simulink model "IBVShandcoded"  (Simulink 5.0)
settings: Solver=ode45  StartTime=0.0  StopTime=30.0  RelTol=1e-3
values from neighbouring files (symbols this model uses):
  c = camera(1000,1000,256,256,512,512)    [initHBVS.m]    (also in vsbrowser.m = handles.c)
  p = reshape(u,2,n)    [CamView.m]    (also in initHBVS.m = polyhedra([0.0 0.0 0; 0.25 0.25 0; -0.25 0.25 0; -0.25 -0.25; vsbrowser.m = handles.p)
  T0c_0 = T0c    [initHBVS.m]
  T0c_x = T0c    [initHBVS.m]
  T0o = handles.T0o    [vsbrowser.m]
undefined symbols (not defined in the file or in its folder): coords, get, GetHMatrix
libraries: vs x10
settings Model: LastModifiedBy=ecervera  BooleanDataType=off

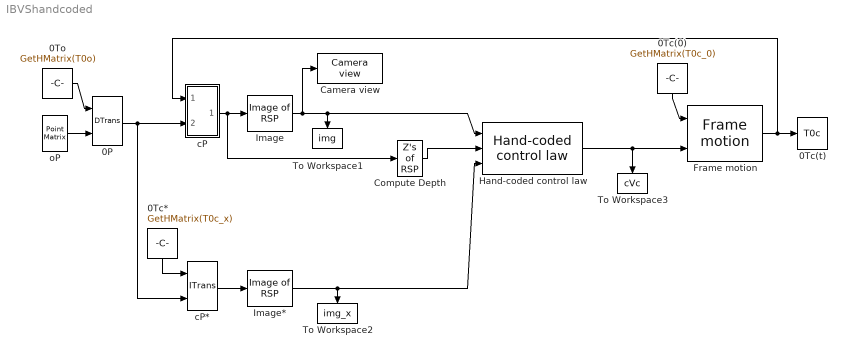
== system IBVShandcoded ==
  0P : vs/Features/DTrans  SimViewingDevice=off  DataTypeOverride=UseLocalSettings  MinMaxOverflowLogging=UseLocalSettings
      settings: Permissions=ReadWrite  RTWFcnNameOpts=Auto  RTWFileNameOpts=Auto
  0Tc(0) : Constant  Orientation=down  Value=GetHMatrix(T0c_0)  VectorParams1D=off
  0Tc(t) : ToWorkspace  VariableName=T0c  SampleTime=-1  SaveFormat=StructureWithTime
  0Tc* : Constant  Orientation=down  Value=GetHMatrix(T0c_x)  VectorParams1D=off
  0To : Constant  Value=GetHMatrix(T0o)  VectorParams1D=off
  Camera view : vs/Camera/Camera view  ms=15  em=normal  umin=0  umax=get(c,'hres')-1  vmin=0  vmax=get(c,'vres')-1  st=-1
  Compute Depth : vs/Features/Z's of RSP  SimViewingDevice=off  DataTypeOverride=UseLocalSettings  MinMaxOverflowLogging=UseLocalSettings
      settings: Permissions=ReadWrite  RTWFcnNameOpts=Auto  RTWFileNameOpts=Auto
  Frame motion : vs/Pose/Frame motion  SimViewingDevice=off  DataTypeOverride=UseLocalSettings  MinMaxOverflowLogging=UseLocalSettings
      settings: Permissions=ReadWrite  RTWFcnNameOpts=Auto  RTWFileNameOpts=Auto
  Hand-coded control law : vs/Jacobian/Hand-coded control law  n=size(coords(p),2)  fu=get(c,'fu')  fv=get(c,'fv')  u0=get(c,'u0')  v0=get(c,'v0')  lambda=lambda
  Image : vs/Camera/Image of RSP  fu=get(c,'fu')  fv=get(c,'fv')  u0=get(c,'u0')  v0=get(c,'v0')
  Image* : vs/Camera/Image of RSP  fu=get(c,'fu')  fv=get(c,'fv')  u0=get(c,'u0')  v0=get(c,'v0')
  To Workspace1 : ToWorkspace  VariableName=img  SampleTime=-1  SaveFormat=StructureWithTime
      settings: Orientation=down
  To Workspace2 : ToWorkspace  VariableName=img_x  SampleTime=-1  SaveFormat=StructureWithTime
      settings: Orientation=down
  To Workspace3 : ToWorkspace  VariableName=cVc  SampleTime=-1  SaveFormat=StructureWithTime
      settings: Orientation=down
  cP : Subsystem  AncestorBlock=vs/Features/ITrans
  cP* : vs/Features/ITrans  SimViewingDevice=off  DataTypeOverride=UseLocalSettings  MinMaxOverflowLogging=UseLocalSettings
      settings: Permissions=ReadWrite  RTWFcnNameOpts=Auto  RTWFileNameOpts=Auto
  oP : vs/Features/Point Matrix  m=coords(p)
  wires:
  oP/1 -> 0P/2
  cP/1(bP) -> Image/1, Compute Depth/1
  Image/1 -> Camera view/1, Hand-coded control law/1, To Workspace1/1
  Frame motion/1 -> 0Tc(t)/1, cP/1(aTb)
  0Tc*/1 -> cP*/1
  cP*/1 -> Image*/1
  Image*/1 -> Hand-coded control law/3, To Workspace2/1
  0Tc(0)/1 -> Frame motion/1
  0To/1 -> 0P/1
  0P/1 -> cP/2(aP), cP*/2
  Hand-coded control law/1 -> To Workspace3/1, Frame motion/2
  Compute Depth/1 -> Hand-coded control law/2

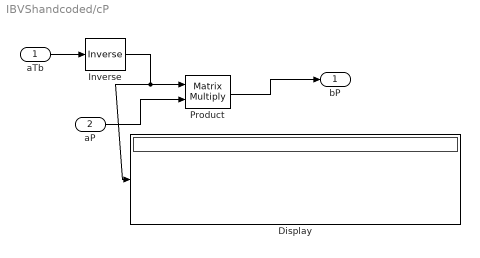
== system IBVShandcoded/cP ==
  aTb : Inport
  aP : Inport  Port=2
  Display : Display
  Inverse : vs/Pose/Inverse
      settings: RTWFcnNameOpts=Auto  RTWFileNameOpts=Auto
  Product : Product  Multiplication=Matrix(*)  SaturateOnIntegerOverflow=on  InputSameDT=on
  bP : Outport
  wires:
  Inverse/1 -> Product/1, Display/1
  aTb/1 -> Inverse/1
  Product/1 -> bP/1
  aP/1 -> Product/2
